simulink model "model"  (R2024a)
settings: Solver=FixedStepAuto  StartTime=0.0  StopTime=80  FixedStep=0.2  RelTol=1e-3
values from neighbouring files (symbols this model uses):
  b = b_V(b_idx)    [experimental_robustness.m]    (also in init.m = 0.3316545; stateFcnTaycan.m = 0.3316545; stateFcnTaycanEKF.m = 0.3316545; test_robustness.m)
  F_max = [22000 1710]    [init.m]    (also in stateFcnTaycan.m = interp1(v_to_F_max_lu, F_max_lu, v, 'linear'); stateFcnTaycanEKF.m = interp1(v_to_F_max_lu, F_max_lu, v, 'linear'))
  F_min = -20000    [init.m]    (also in stateFcnTaycan.m; stateFcnTaycanEKF.m)
  g = 9.81    [init.m]
  m = m_V(m_idx)    [experimental_robustness.m]    (also in init.m = 2140; run_mpc_vs_pid_robustness_test.m; stateFcnTaycan.m = 2140; stateFcnTaycanEKF.m = 2140)
  Ts = 1    [init.m]    (also in stateFcnTaycanEKF.m = uk(3))
  v_to_F_max = [0 72]    [init.m]
libraries: simulink x3, sharedTrackingLibrary x1, mpclib x1
settings Model: Creator=berto  LastModifiedBy=berto
settings SolverCC: MinimalZcImpactIntegration=on

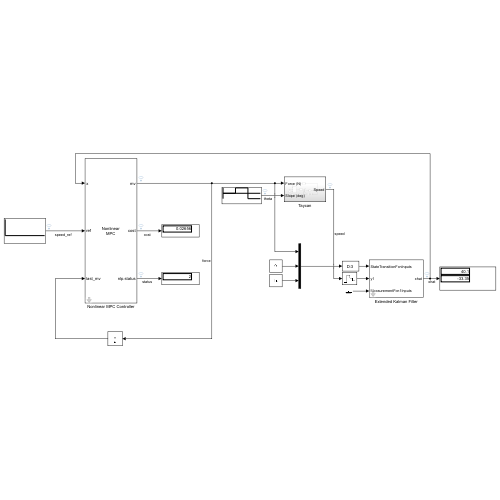
[thumbnail: Simulink's stored preview of the top-level diagram]
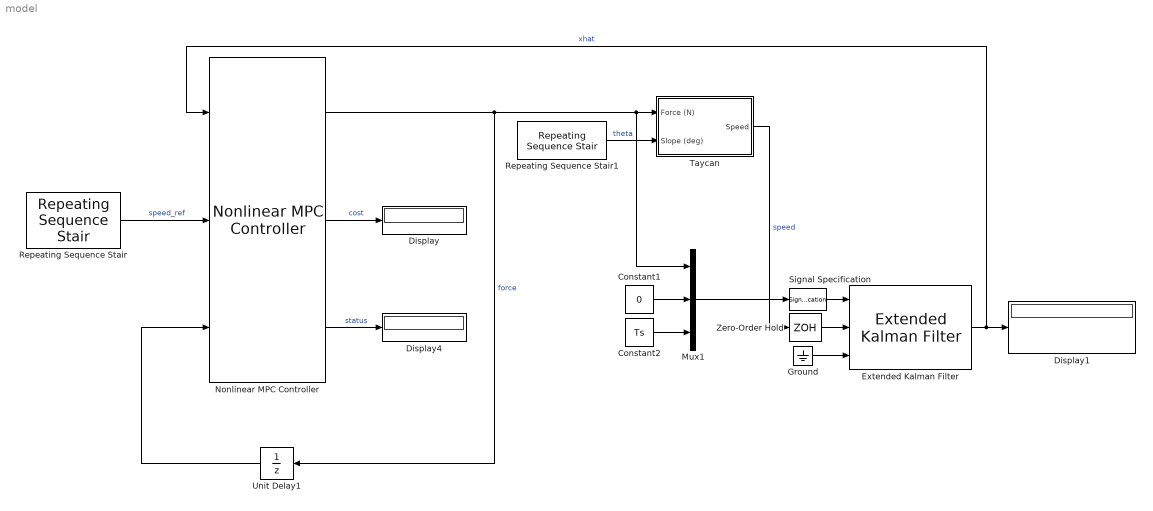
== system model ==
  Constant1 : Constant  Value=0
  Constant2 : Constant  Value=Ts
  Display : Display
  Display1 : Display
  Display4 : Display
  Extended Kalman Filter : sharedTrackingLibrary/Extended Kalman Filter  StateTransitionFcn=stateFcnTaycanEKF  HasStateTransitionJacobianFcn=off  HasAdditiveProcessNoise=Additive  ProcessNoise=diag([0 1e5])  HasTimeVaryingProcessNoise=off  HasStateTransitionFcnExtraArgument=1  InitialState=[0; 0]  InitialStateCovariance=diag([1 100])  MeasurementFcn1=outputFcnTaycan  HasMeasurementJacobianFcn1=off  HasMeasurementEnablePort1=off  HasAdditiveMeasurementNoise1=Additive  MeasurementNoise1=1  HasTimeVaryingMeasurementNoise1=off  HasMeasurementFcnExtraArgument1=1  HasMeasurementWrapping1=off  MeasurementFcn2=myMeasurementFcn  HasMeasurementJacobianFcn2=off  HasMeasurementEnablePort2=off  HasAdditiveMeasurementNoise2=Additive  MeasurementNoise2=1  HasTimeVaryingMeasurementNoise2=off  HasMeasurementFcnExtraArgument2=0  HasMeasurementWrapping2=off  MeasurementFcn3=myMeasurementFcn  HasMeasurementJacobianFcn3=off  HasMeasurementEnablePort3=off  HasAdditiveMeasurementNoise3=Additive  MeasurementNoise3=1  HasTimeVaryingMeasurementNoise3=off  HasMeasurementFcnExtraArgument3=0  HasMeasurementWrapping3=off  MeasurementFcn4=myMeasurementFcn  HasMeasurementJacobianFcn4=off  HasMeasurementEnablePort4=off  HasAdditiveMeasurementNoise4=Additive  MeasurementNoise4=1  HasTimeVaryingMeasurementNoise4=off  HasMeasurementFcnExtraArgument4=0  HasMeasurementWrapping4=off  MeasurementFcn5=myMeasurementFcn  HasMeasurementJacobianFcn5=off  HasMeasurementEnablePort5=off  HasAdditiveMeasurementNoise5=Additive  MeasurementNoise5=1  HasTimeVaryingMeasurementNoise5=off  HasMeasurementFcnExtraArgument5=0  HasMeasurementWrapping5=off  EnableMultirate=off  StateTransitionFcnSampleTime=1  MeasurementFcn1SampleTime=1  MeasurementFcn2SampleTime=1  MeasurementFcn3SampleTime=1  MeasurementFcn4SampleTime=1  MeasurementFcn5SampleTime=1  UseCurrentEstimator=on  OutputStateCovariance=off  DataType=double  SampleTime=Ts  NumberOfMeasurements=1
  Ground : Ground
  Mux1 : Mux  Inputs=3
  Nonlinear MPC Controller : mpclib/Nonlinear MPC Controller  nlmpcobj=nlobj  UseObjectTs=on  UseMEX=off  md_enabled=off  mvtarget_enabled=off  param_enabled=off  cost_enabled=on  mvseq_enabled=off  stateseq_enabled=off  ovseq_enabled=off  slack_enabled=off  status_enabled=on  ov_min=off  ov_max=off  mv_min=off  mv_max=off  mvrate_min=off  mvrate_max=off  state_min=off  state_max=off  ov_weight=off  mv_weight=off  mvrate_weight=off  ecr_weight=off  nlp_initialize=off
  Repeating Sequence Stair : simulink/Sources/Repeating Sequence Stair  OutValues=40  tsamp=20  OutMin=[]  OutMax=[]  OutDataTypeStr=double  OutputDataTypeScalingMode=double  OutDataType=fixdt(0,8)  ConRadixGroup=Best Precision: Vector-wise  OutScaling=2^-12
  Repeating Sequence Stair1 : simulink/Sources/Repeating Sequence Stair  OutValues=[0 10 -10].'  tsamp=20  OutMin=[]  OutMax=[]  OutDataTypeStr=double  OutputDataTypeScalingMode=double  OutDataType=fixdt(0,8)  ConRadixGroup=Best Precision: Vector-wise  OutScaling=2^-12
  Signal Specification : SignalSpecification  Dimensions=3
  Taycan : Subsystem
  Unit Delay1 : UnitDelay  SampleTime=Ts  HasFrameUpgradeWarning=on
  Zero-Order Hold : ZeroOrderHold  SampleTime=Ts
  wires:
  Taycan/1(Speed) -> Zero-Order Hold/1  "speed"
  Nonlinear MPC Controller/1 -> Taycan/1(Force (N)), Mux1/1, Unit Delay1/1  "force"
  Repeating Sequence Stair/1 -> Nonlinear MPC Controller/2  "speed_ref"
  Unit Delay1/1 -> Nonlinear MPC Controller/3
  Nonlinear MPC Controller/2 -> Display/1  "cost"
  Nonlinear MPC Controller/3 -> Display4/1  "status"
  Repeating Sequence Stair1/1 -> Taycan/2(Slope (deg))  "theta"
  Constant1/1 -> Mux1/2
  Extended Kalman Filter/1 -> Display1/1, Nonlinear MPC Controller/1  "xhat"
  Zero-Order Hold/1 -> Extended Kalman Filter/2
  Mux1/1 -> Signal Specification/1
  Signal Specification/1 -> Extended Kalman Filter/1
  Constant2/1 -> Mux1/3
  Ground/1 -> Extended Kalman Filter/3

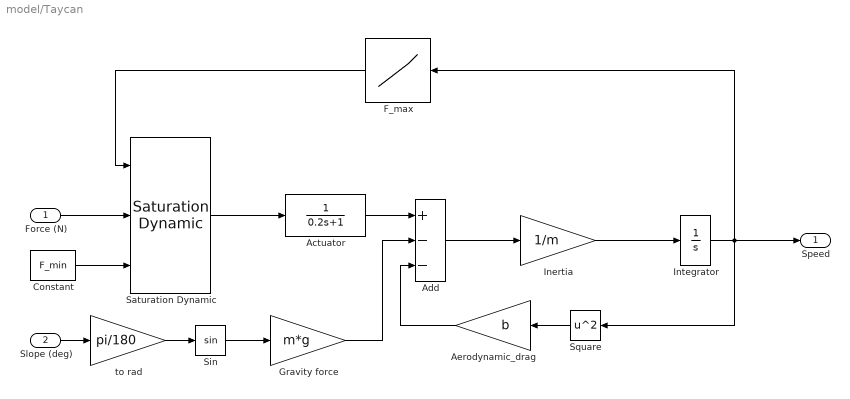
== system model/Taycan ==
  Force (N) : Inport
  Slope (deg) : Inport  Port=2
  Actuator : TransferFcn  Denominator=[0.2 1]
  Add : Sum  Inputs=+--
  Aerodynamic_drag : Gain  Gain=b
  Constant : Constant  Value=F_min
  F_max : Lookup_n-D  NumberOfTableDimensions=1  BreakpointsForDimension1=v_to_F_max  Table=F_max  ExtrapMethod=Clip  InternalRulePriority=Speed  RndMeth=Simplest
  Gravity force : Gain  Gain=m*g
  Inertia : Gain  Gain=1/m
  Integrator : Integrator
  Saturation Dynamic : simulink/Discontinuities/Saturation Dynamic  OutMin=[]  OutMax=[]  OutDataTypeStr=Inherit: Same as second input  OutDataType=fixdt(1, 16)  OutScaling=2^-10  DoSatur=off
  Sin : Trigonometry
  Square : Math  Operator=square
  to rad : Gain  Gain=pi/180
  Speed : Outport
  wires:
  Force (N)/1 -> Saturation Dynamic/2
  Actuator/1 -> Add/1
  Integrator/1 -> F_max/1, Speed/1, Square/1
  Constant/1 -> Saturation Dynamic/3
  Saturation Dynamic/1 -> Actuator/1
  F_max/1 -> Saturation Dynamic/1
  Aerodynamic_drag/1 -> Add/3
  Add/1 -> Inertia/1
  Inertia/1 -> Integrator/1
  Square/1 -> Aerodynamic_drag/1
  Slope (deg)/1 -> to rad/1
  Sin/1 -> Gravity force/1
  Gravity force/1 -> Add/2
  to rad/1 -> Sin/1
